simulink model "modeloNoLineal"  (Simulink 7.9)
settings: Solver=ode45  StartTime=0.0  StopTime=900.0  RelTol=1e-3
settings Model: Creator=root  LastModifiedBy=root

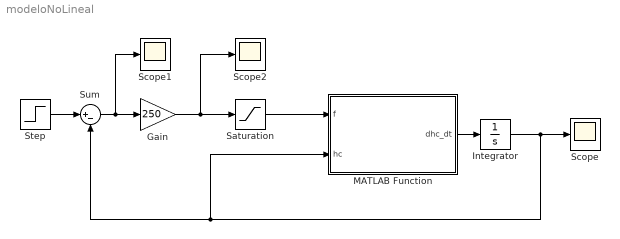
== system modeloNoLineal ==
  Gain : Gain  Gain=250
  Integrator : Integrator  InitialCondition=10  UpperSaturationLimit=70  LowerSaturationLimit=0
  MATLAB Function : MATLAB Function  TreatAsAtomicUnit=on
  Saturation : Saturate  UpperLimit=100  LowerLimit=0
  Scope : Scope
  Scope1 : Scope
  Scope2 : Scope
      settings: SaveName=ScopeData2
  Step : Step  After=20  SampleTime=0
  Sum : Sum  Inputs=|+-
  wires:
  Integrator/1 -> MATLAB Function/2(hc), Sum/2, Scope/1
  Gain/1 -> Scope2/1, Saturation/1
  Sum/1 -> Gain/1, Scope1/1
  Step/1 -> Sum/1
  Saturation/1 -> MATLAB Function/1(f)
  MATLAB Function/1(dhc_dt) -> Integrator/1

== matlab function MATLAB Function ==
  data: f input double; dhc_dt output double; hc input double
function dhc_dt = ModeloNoLineal(f, hc)
%#codegen

    dhc_dt = (5.43*f-78.43-20.21*sqrt(abs(hc)))/(0.63*(hc.^2)+11.4*hc+17.1);
end
